simulink model "threephase_power_inverter"  (R2014a)
settings: Solver=ode23tb  StartTime=0.0  StopTime=0.2  RelTol=1e-4
StartFcn:
  | tic;
StopFcn:
  | toc;
libraries: powerlib x6, powerlib_meascontrol x1
settings Model: Creator=schandra  LastModifiedBy=cosorio
settings DataIOCC: SaveOutput=off  SignalLogging=off  DSMLogging=off  SaveTime=off
settings DebuggingCC: UnderspecifiedInitializationDetection=Classic  SolverPrmCheckMsg=none

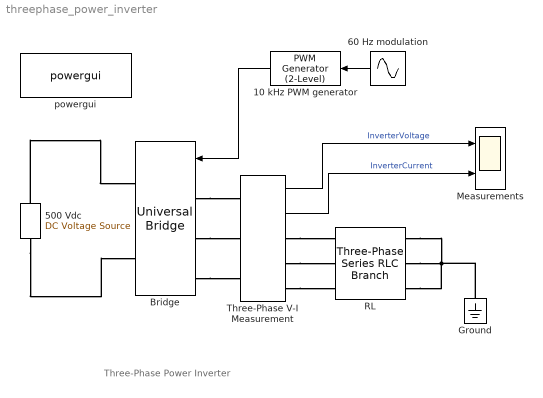
== system threephase_power_inverter ==
  note: Three-Phase Power Inverter
  10 kHz PWM generator : powerlib_meascontrol/Pulse & Signal Generators/PWM Generator (2-Level)  ModulatorType=Three-phase bridge (6 pulses)  ModulatorMode=Unsynchronized  nF=27  Fc=10000  ModulatingSignals=off  m=0.8  Freq=60  Phase=0  Ts=1e-6
  500 Vdc : powerlib/Electrical Sources/DC Voltage Source  Amplitude=500  Measurements=None
  60 Hz modulation : Sin  Frequency=60*2*pi  Phase=[0, 120*pi/180, -120*pi/180]  SampleTime=1e-4
  Bridge : powerlib/Power Electronics/Universal Bridge  Arms=3  SnubberResistance=1e5  SnubberCapacitance=inf  Device=IGBT / Diodes  Ron=1e-4  Lon=0  ForwardVoltages="[  0  0  ]"  ForwardVoltage=0  GTOparameters=[ 10e-6 , 20e-6 ]  IGBTparameters=[ 1e-6 , 2e-6 ]  Measurements=None  Measurements_2=None  converterType=Rectifier
      settings: AttributesFormatString=|
      | %<Device>
      | three arms
      | 6 devices
  Ground : powerlib/Elements/Ground  LConnTagsString=a
  Measurements : Scope  NumInputPorts=2
      settings: YMin=-400~-300  YMax=400~300  SaveName=InverterData
  RL : powerlib/Elements/Three-Phase Series RLC Branch  LConnTagsString=A|B|C  RConnTagsString=A|B|C  BranchType=RL  Resistance=1  Inductance=1e-3  Capacitance=1e-6  Measurements=None
  Three-Phase V-I Measurement : powerlib/Measurements/Three-Phase V-I Measurement  VoltageMeasurement=phase-to-ground  SetLabelV=off  LabelV=Vabc  Vpu=off  VpuLL=off  CurrentMeasurement=yes  SetLabelI=off  LabelI=Iabc  Ipu=off  Pbase=100e6  Vbase=500e3  OutputType=Complex  PhasorSimulation=off  PSBequivalent=0
  powergui : powerlib/powergui  Priority=1  SimulationMode=Discrete  SolverType=Tustin  SampleTime=1e-6  frequency=60  SPID=off  DisableSnubberDevices=on  DisableRonSwitches=on  DisableVfSwitches=off  SwTol=0  Interpol=off  DisplayEquations=off  Ts=0  methode=off  frequencyindice=0  Pbase=100e6  ErrMax=1e-4  Iterations=50  UnitsV=kV  UnitsW=MW  FunctionMessages=off  echomessages=off  HookPort=off  EnableUseOfTLC=off  x0status=blocks  RestoreLinks=warning  ResistiveCurrentMeasurement=off  Frange=[0:2:500]  Ylog=off  Xlog=on  ShowGrid=off  save=off  variable=ZData  structure=InverterData  ZoomFFT=off  StartTime=0.05  cycles=2  DisplayStyle=1  fundamental=60  FreqAxis=on  MaxFrequency=10000  frequencyindicesteady=1  RmsSteady=1  display=off
  wires:
  60 Hz modulation/1 -> 10 kHz PWM generator/1
  Three-Phase V-I Measurement/2 -> Measurements/2  "InverterCurrent"
  Three-Phase V-I Measurement/1 -> Measurements/1  "InverterVoltage"
  10 kHz PWM generator/1 -> Bridge/1
  connections:
  Ground/LConn1 -- RL/RConn3 -- RL/RConn1 -- RL/RConn2
  Three-Phase V-I Measurement/RConn1 -- RL/LConn1
  Three-Phase V-I Measurement/RConn2 -- RL/LConn2
  Three-Phase V-I Measurement/RConn3 -- RL/LConn3
  500 Vdc/LConn1 -- Bridge/RConn2
  500 Vdc/RConn1 -- Bridge/RConn1
  Bridge/LConn3 -- Three-Phase V-I Measurement/LConn3
  Bridge/LConn2 -- Three-Phase V-I Measurement/LConn2
  Bridge/LConn1 -- Three-Phase V-I Measurement/LConn1
